simulink library "squareWave_ul"  (R2020a)
settings: Solver=VariableStepAuto  StartTime=0.0  StopTime=10.0  RelTol=1e-3
settings Model: Creator=Ayaz  LastModifiedBy=Ayaz

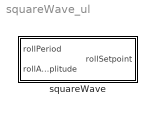
== system squareWave_ul ==
  squareWave : Subsystem  mask{startDelay=4}
      mask prompts: startDelay "Square wave initialization dealy: values*rollPeriod"
      mask TypeOptions startDelay: Gain/Gain

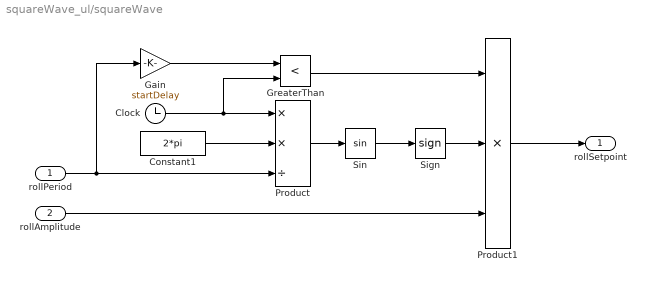
== system squareWave_ul/squareWave ==
  rollPeriod : Inport
  rollAmplitude : Inport  Port=2
  Clock : Clock
  Constant1 : Constant  Value=2*pi
  Gain : Gain  Gain=startDelay
  GreaterThan : RelationalOperator  Operator=<  OutDataTypeStr=boolean  RndMeth=Simplest
  Product : Product  Inputs=**/
  Product1 : Product  Inputs=3
  Sign : Signum
  Sin : Trigonometry
  rollSetpoint : Outport
  wires:
  Constant1/1 -> Product/2
  rollPeriod/1 -> Gain/1, Product/3
  Sign/1 -> Product1/2
  Sin/1 -> Sign/1
  Clock/1 -> GreaterThan/2, Product/1
  Product/1 -> Sin/1
  rollAmplitude/1 -> Product1/3
  Product1/1 -> rollSetpoint/1
  Gain/1 -> GreaterThan/1
  GreaterThan/1 -> Product1/1
